simulink model "mIpCLwindy_wind_rsw"  (R2018b)
settings: Solver=ode45  StartTime=0.0  StopTime=30  RelTol=1e-3
values from neighbouring files (symbols this model uses):
  Ac = Ad - Ld*Cd -Bd*Kd    [sol_wind_rsw.m]
  ADxx = Axx*Dxx    (= 3.3896759392e-07)    [miParameters_rsw_final.m]    (also in mipParameters.m; mipParameters_rsw.m; sol_wind_rsw.m)
  AFxx = Axx*Fxx    (= 2.38487861376e-07)    [miParameters_rsw_final.m]    (also in mipParameters.m; mipParameters_rsw.m; sol_wind_rsw.m)
  Ao = Ad - Ld*Cd    [sol_wind_rsw.m]
  Axx = Ib + mb*l*l    (= 0.000740848)    [miParameters_rsw_final.m]    (also in mipParameters.m; mipParameters_rsw.m; sol_wind_rsw.m)
  Bc = Ld    [sol_wind_rsw.m]
  BDxx = Bxx*Dxx    (= 4.24968093432e-05)    [miParameters_rsw_final.m]    (also in mipParameters.m; mipParameters_rsw.m; sol_wind_rsw.m)
  BExx = Bxx*Exx    (= 2.9899534225e-05)    [miParameters_rsw_final.m]    (also in mipParameters.m; mipParameters_rsw.m; sol_wind_rsw.m)
  Bo = [Bd Ld]    [sol_wind_rsw.m]
  Cc = [-Kd; eye(6,6)]    [sol_wind_rsw.m]
  CExx = Cxx*Exx    (= 1.03627335744e-07)    [miParameters_rsw_final.m]    (also in mipParameters.m; mipParameters_rsw.m; sol_wind_rsw.m)
  CFxx = Cxx*Fxx    (= 1.03627335744e-07)    [miParameters_rsw_final.m]    (also in mipParameters.m; mipParameters_rsw.m; sol_wind_rsw.m)
  Co = eye(6)    [sol_wind_rsw.m]
  Cxx = mb*r*l    (= 0.000321912)    [miParameters_rsw_final.m]    (also in mipParameters.m; mipParameters_rsw.m; sol_wind_rsw.m)
  Dc = zeros(7, 2)    [sol_wind_rsw.m]
  Do = zeros(6,3)    [sol_wind_rsw.m]
  Dxx = Iw+(mw+mb)*r*r    (= 0.00045754)    [miParameters_rsw_final.m]    (also in mipParameters.m; mipParameters_rsw.m; sol_wind_rsw.m)
  Exx = Cxx    (= 0.000321912)    [miParameters_rsw_final.m]    (also in mipParameters.m; mipParameters_rsw.m; sol_wind_rsw.m)
  ktL = 32.0130    (= 32.013)    [miParameters_rsw_final.m]    (also in mipParameters.m; mipParameters_rsw.m; sol_wind_rsw.m)
  kvktL = 6.4697    [miParameters_rsw_final.m]    (also in mipParameters.m; mipParameters_rsw.m; sol_wind_rsw.m)
  RL = 1500    [miParameters_rsw_final.m]    (also in mipParameters.m; mipParameters_rsw.m; sol_wind_rsw.m)
  Ts = 1/200    (= 0.005)    [miParameters_rsw_final.m]    (also in mipParameters.m; mipParameters_rsw.m; sol_rsw.m; sol_wind_rsw.m)
libraries: simulink x2
settings Model: Creator=bob  LastModifiedBy=Administrator
settings DataIOCC: LimitDataPoints=on  SaveFormat=Array
settings OptimizationCC: BlockReduction=off  BooleanDataType=off  LifeSpan=inf
settings DebuggingCC: SaveWithParameterizedLinksMsg=none  UnderspecifiedInitializationDetection=Classic  MergeDetectMultiDrivingBlocksExec=none  SignalResolutionControl=TryResolveAllWithWarning  SFUnexpectedBacktrackingDiag=warning  SFNoUnconditionalDefaultTransitionDiag=warning  SFExecutionAtInitializationDiag=none
settings HardwareCC: ProdBitPerPointer=32  ProdBitPerSizeT=32  ProdBitPerPtrDiffT=32  ProdLargestAtomicFloat=None  ProdIntDivRoundTo=Undefined  ProdEndianess=Unspecified  ProdWordSize=32  ProdHWDeviceType=32-bit Generic  TargetUnknown=on
settings ModelReferenceCC: PropagateSignalLabelsOutOfModel=off
settings SFSimCC: SimUseLocalCustomCode=off
settings RTWCC: RTWUseLocalCustomCode=off
settings CodeAppCC: StateflowObjectComments=on
settings GRTTargetCC: TargetLangStandard=C89/C90 (ANSI)  GeneratePreprocessorConditionals=Disable all
settings ConfigComp: CovMetricSettings=dw  CovHtmlReporting=on  CovSaveCumulativeToWorkspaceVar=on  CovSaveSingleToWorkspaceVar=on  CovExternalEMLEnable=off  CovSFcnEnable=off

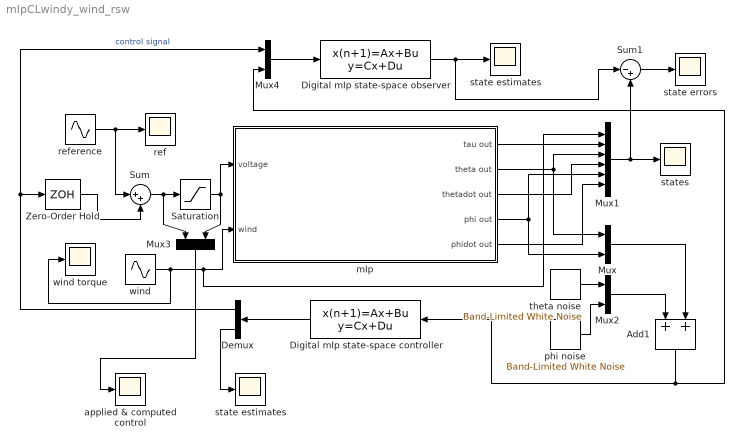
== system mIpCLwindy_wind_rsw ==
  Add1 : Sum  Inputs=2
  Demux : Demux  Outputs=[1 6]
  Digital mIp state-space controller : DiscreteStateSpace  A=Ac  B=Bc  C=Cc  D=Dc  SampleTime=Ts
  Digital mIp state-space observer : DiscreteStateSpace  A=Ao  B=Bo  C=Co  D=Do  SampleTime=Ts
  Mux{,2..4} (4 alike) : Mux  Inputs=2
  Mux1 : Mux  Inputs=6
  Saturation : Saturate  UpperLimit=6  LowerLimit=-6
  Sum : Sum  Inputs=|++
  Sum1 : Sum  Inputs=|-+
  Zero-Order Hold : ZeroOrderHold  Tag=zero-order hold  SampleTime=-1
  applied & computed control : Scope
  mIp : Subsystem
  phi noise : simulink/Sources/Band-Limited White Noise  Cov=0  Ts=Ts  seed=[23341]
  ref : Scope
  reference : Sin  Amplitude=0
  state errors : Scope
  state estimates : Scope
  "state estimates " : Scope
  states : Scope
  theta noise : simulink/Sources/Band-Limited White Noise  Cov=0  Ts=Ts  seed=[23341]
  wind : Sin  Amplitude=0  Bias=2  SampleTime=0
  wind torque : Scope
  wires:
  mIp/2(theta out) -> Mux1/3, Mux/1
  mIp/4(phi out) -> Mux1/5, Mux/2
  mIp/1(tau out) -> Mux1/2
  mIp/5(phidot out) -> Mux1/6
  Mux1/1 -> Sum1/2, states/1
  phi noise/1 -> Mux2/2
  Mux2/1 -> Add1/1
  Mux/1 -> Add1/2
  Add1/1 -> Mux4/2, Digital mIp state-space controller/1
  Saturation/1 -> Mux3/2, mIp/1(voltage)
  Digital mIp state-space controller/1 -> Demux/1
  Demux/1 -> Mux4/1, Zero-Order Hold/1  "control signal"
  Mux3/1 -> applied & computed control/1
  wind/1 -> wind torque/1, Mux1/1, mIp/2(wind)
  reference/1 -> ref/1, Sum/1
  Zero-Order Hold/1 -> Sum/2
  Sum/1 -> Mux3/1, Saturation/1
  Digital mIp state-space observer/1 -> Sum1/1, state estimates/1
  Mux4/1 -> Digital mIp state-space observer/1
  theta noise/1 -> Mux2/1
  Demux/2 -> "state estimates "/1
  mIp/3(thetadot out) -> Mux1/4
  Sum1/1 -> state errors/1

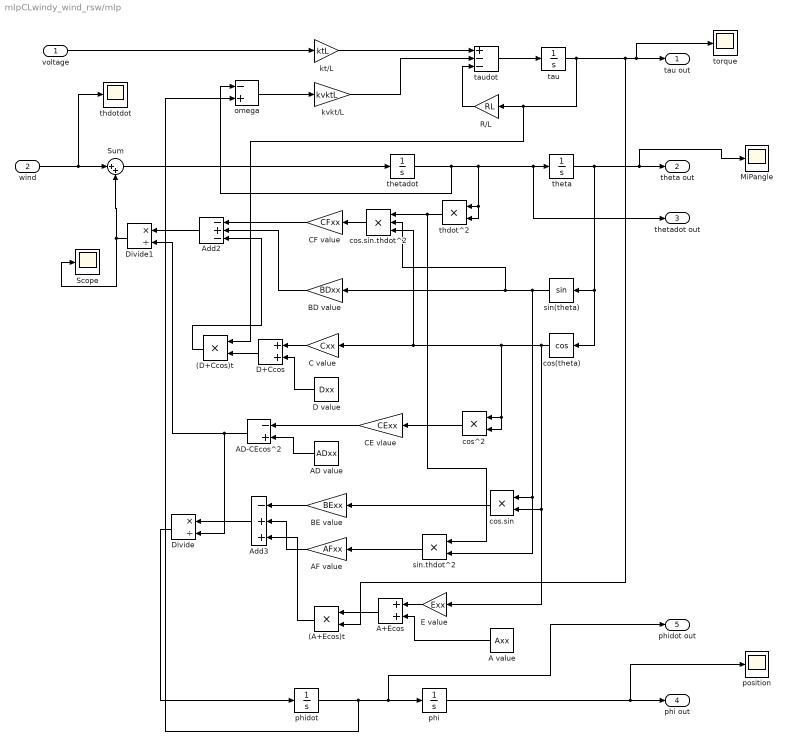
== system mIpCLwindy_wind_rsw/mIp ==
  voltage : Inport
  wind : Inport  Port=2
  (A+Ecos)t : Product
  (D+Ccos)t : Product
  A value : Constant  Value=Axx
  A+Ecos : Sum  Inputs=2
  AD value : Constant  Value=ADxx
  AD-CEcos^2 : Sum  Inputs=-+
  AF value : Gain  Gain=AFxx
  Add2 : Sum  Inputs=-+-
  Add3 : Sum  Inputs=-++
  BD value : Gain  Gain=BDxx
  BE value : Gain  Gain=BExx
  C value : Gain  Gain=Cxx
  CE vlaue : Gain  Gain=CExx
  CF value : Gain  Gain=CFxx
  D value : Constant  Value=Dxx
  D+Ccos : Sum
  Divide : Product  Inputs=*/
  Divide1 : Product  Inputs=*/
  E value : Gain  Gain=Exx
  MiPangle : Scope
  R/L : Gain  Gain=RL
  Scope : Scope
  Sum : Sum  Inputs=|++
  cos(theta) : Trigonometry  Operator=cos
  cos.sin : Product
  cos.sin.thdot^2 : Product  Inputs=3
  cos^2 : Product
  kt/L : Gain  Gain=ktL
  kvkt/L : Gain  Gain=kvktL
  omega : Sum  Inputs=-+
  phi : Integrator
  phidot : Integrator
  position : Scope
  "sin(theta) " : Trigonometry
  sin.thdot^2 : Product
  tau : Integrator
  taudot : Sum  Inputs=+--
  thdot^2 : Product
  "thdotdot " : Scope
  theta : Integrator
  thetadot : Integrator
  torque : Scope
  tau out : Outport
  theta out : Outport  Port=2
  thetadot out : Outport  Port=3
  phi out : Outport  Port=4
  phidot out : Outport  Port=5
  wires:
  R/L/1 -> taudot/3
  voltage/1 -> kt/L/1
  kt/L/1 -> taudot/1
  taudot/1 -> tau/1
  kvkt/L/1 -> taudot/2
  omega/1 -> kvkt/L/1
  phi/1 -> position/1, phi out/1
  cos(theta)/1 -> E value/1, cos.sin/2, cos^2/2, cos^2/1, C value/1, cos.sin.thdot^2/3
  "sin(theta) "/1 -> sin.thdot^2/2, cos.sin/1, cos.sin.thdot^2/2, BD value/1
  thetadot/1 -> omega/1, thdot^2/2, thdot^2/1, thetadot out/1, theta/1
  thdot^2/1 -> sin.thdot^2/1, cos.sin.thdot^2/1
  cos.sin.thdot^2/1 -> CF value/1
  cos^2/1 -> CE vlaue/1
  CE vlaue/1 -> AD-CEcos^2/1
  AD value/1 -> AD-CEcos^2/2
  C value/1 -> D+Ccos/1
  D value/1 -> D+Ccos/2
  D+Ccos/1 -> (D+Ccos)t/2
  tau/1 -> (A+Ecos)t/2, torque/1, tau out/1, (D+Ccos)t/1, R/L/1
  CF value/1 -> Add2/1
  BD value/1 -> Add2/2
  (D+Ccos)t/1 -> Add2/3
  Add2/1 -> Divide1/1
  AD-CEcos^2/1 -> Divide/2, Divide1/2
  Divide1/1 -> Scope/1, Sum/2
  cos.sin/1 -> BE value/1
  sin.thdot^2/1 -> AF value/1
  E value/1 -> A+Ecos/1
  A value/1 -> A+Ecos/2
  A+Ecos/1 -> (A+Ecos)t/1
  theta/1 -> MiPangle/1, theta out/1, cos(theta)/1, "sin(theta) "/1
  BE value/1 -> Add3/1
  AF value/1 -> Add3/2
  (A+Ecos)t/1 -> Add3/3
  Add3/1 -> Divide/1
  Divide/1 -> phidot/1
  phidot/1 -> omega/2, phidot out/1, phi/1
  wind/1 -> "thdotdot "/1, Sum/1
  Sum/1 -> thetadot/1
